simulink model "a1"  (Simulink 5.0)
settings: Solver=ode45  SolverMode=SingleTasking  StartTime=0.0  StopTime=1  RelTol=1e-4  AbsTol=1e-8
CloseFcn:
  | ;slview('closediagram',bdroot);
settings Model: LastModifiedBy=Âlue Phoenix  LimitDataPoints=off  BlockReductionOpt=off  BooleanDataType=off

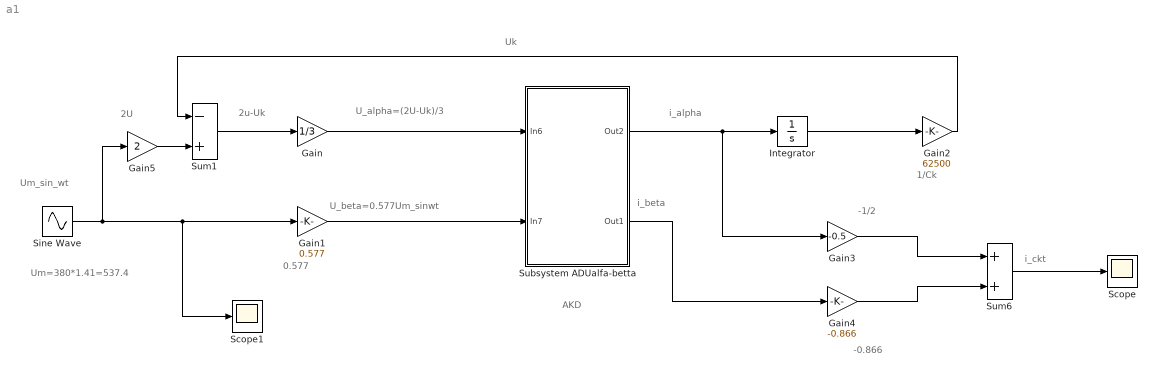
== system a1 ==
  note: U_alpha=(2U-Uk)/3
  note: Uk
  note: i_alpha
  note: i_beta
  note: 1/Ck
  note: -1/2
  note: -0.866
  note: i_ckt
  note: AKD
  note: Um_sin_wt
  note: Um=380*1.41=537.4
  note: 0.577
  note: 2U
  note: U_beta=0.577Um_sinwt
  note: 2u-Uk
  Gain : Gain  Gain=1/3  SaturateOnIntegerOverflow=on
  Gain1 : Gain  Gain=0.577  SaturateOnIntegerOverflow=on
  Gain2 : Gain  Gain=62500  SaturateOnIntegerOverflow=on
  Gain3 : Gain  Gain=-0.5  SaturateOnIntegerOverflow=on
  Gain4 : Gain  Gain=-0.866  SaturateOnIntegerOverflow=on
  Gain5 : Gain  Gain=2  SaturateOnIntegerOverflow=on
  Integrator : Integrator
  Scope : Scope
      settings: SaveName=ScopeData2
  Scope1 : Scope
      settings: SaveName=ScopeData3
  Sine Wave : Sin  Amplitude=537.4  Frequency=314  SampleTime=0
  Subsystem ADUalfa-betta : Subsystem
  Sum1 : Sum  Inputs=-+  SaturateOnIntegerOverflow=on  InputSameDT=on
  Sum6 : Sum  SaturateOnIntegerOverflow=on  InputSameDT=on
  wires:
  Sum1/1 -> Gain/1
  Gain/1 -> Subsystem ADUalfa-betta/1(In6)
  Gain1/1 -> Subsystem ADUalfa-betta/2(In7)
  Sine Wave/1 -> Gain1/1, Scope1/1, Gain5/1
  Subsystem ADUalfa-betta/1(Out2) -> Integrator/1, Gain3/1
  Integrator/1 -> Gain2/1
  Gain3/1 -> Sum6/1
  Gain4/1 -> Sum6/2
  Subsystem ADUalfa-betta/2(Out1) -> Gain4/1
  Gain2/1 -> Sum1/1
  Sum6/1 -> Scope/1
  Gain5/1 -> Sum1/2

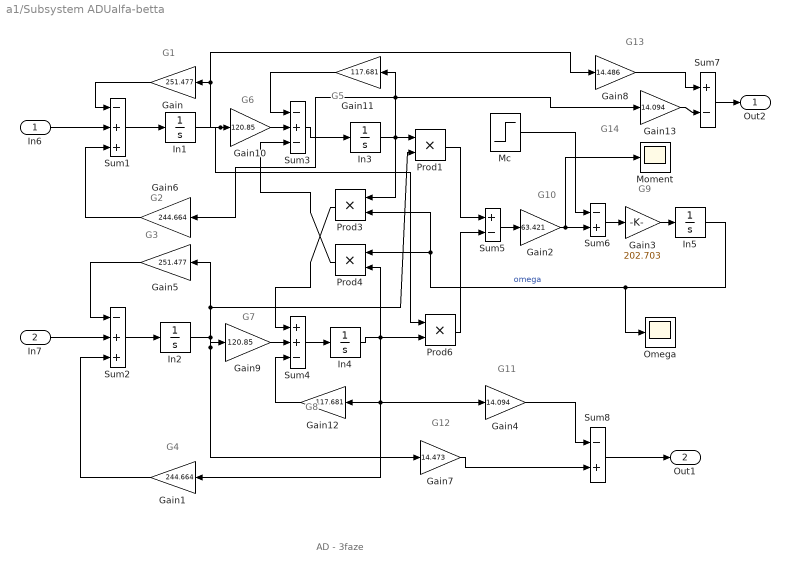
== system a1/Subsystem ADUalfa-betta ==
  note: G1
  note: G2
  note: G3
  note: G4
  note: G10
  note: G9
  note: G6
  note: G7
  note: G8
  note: G5
  note: AD - 3faze
  note: G14
  note: G12
  note: G13
  note: G11
  In6 : Inport
  In7 : Inport  Port=2
  "  Prod1" : Product  SaturateOnIntegerOverflow=on  InputSameDT=on
  Gain : Gain  Orientation=left  Gain=251.477  SaturateOnIntegerOverflow=on
  Gain1 : Gain  Orientation=left  Gain=244.664  SaturateOnIntegerOverflow=on
  Gain10 : Gain  Gain=120.85  SaturateOnIntegerOverflow=on
  Gain11 : Gain  Orientation=left  Gain=117.681  SaturateOnIntegerOverflow=on
  Gain12 : Gain  Orientation=left  Gain=117.681  SaturateOnIntegerOverflow=on
  Gain13 : Gain  Gain=14.094  SaturateOnIntegerOverflow=on
  Gain2 : Gain  Gain=63.421  SaturateOnIntegerOverflow=on
  Gain3 : Gain  Gain=202.703  SaturateOnIntegerOverflow=on
  Gain4 : Gain  Gain=14.094  SaturateOnIntegerOverflow=on
  Gain5 : Gain  Orientation=left  Gain=251.477  SaturateOnIntegerOverflow=on
  Gain6 : Gain  Orientation=left  Gain=244.664  SaturateOnIntegerOverflow=on
  Gain7 : Gain  Gain=14.473  SaturateOnIntegerOverflow=on
  Gain8 : Gain  Gain=14.486  SaturateOnIntegerOverflow=on
  Gain9 : Gain  Gain=120.85  SaturateOnIntegerOverflow=on
  In{1..5} (5 alike) : Integrator
  Mc : Step  Time=0.1  Before=0.0  After=17  SampleTime=0
  Moment : Scope
      settings: TickLabels=on  TimeRange=1  YMin=-10  YMax=20  DataFormat=Array
  Omega : Scope
      settings: TickLabels=on  TimeRange=0.5  YMin=0  YMax=1000  DataFormat=Array
  Prod3 : Product  Orientation=left  SaturateOnIntegerOverflow=on  InputSameDT=on
  Prod4 : Product  Orientation=left  SaturateOnIntegerOverflow=on  InputSameDT=on
  Prod6 : Product  SaturateOnIntegerOverflow=on  InputSameDT=on
  Sum1 : Sum  Inputs=-++  SaturateOnIntegerOverflow=on  InputSameDT=on
  Sum2 : Sum  Inputs=-++  SaturateOnIntegerOverflow=on  InputSameDT=on
  Sum3 : Sum  Inputs=-+-  SaturateOnIntegerOverflow=on  InputSameDT=on
  Sum4 : Sum  Inputs=++-  SaturateOnIntegerOverflow=on  InputSameDT=on
  Sum5 : Sum  Inputs=+-  SaturateOnIntegerOverflow=on  InputSameDT=on
  Sum6 : Sum  Inputs=-+  SaturateOnIntegerOverflow=on  InputSameDT=on
  Sum7 : Sum  Inputs=+-  SaturateOnIntegerOverflow=on  InputSameDT=on
  Sum8 : Sum  Inputs=-+  SaturateOnIntegerOverflow=on  InputSameDT=on
  Out2 : Outport
  Out1 : Outport  Port=2
  wires:
  Gain/1 -> Sum1/1
  Sum2/1 -> In2/1
  In4/1 -> Prod4/2, Prod6/2, Gain1/1, Gain12/1, Gain4/1
  In3/1 -> Prod3/1, "  Prod1"/1, Gain6/1, Gain11/1, Gain13/1
  Prod6/1 -> Sum5/2
  Sum6/1 -> Gain3/1
  Gain3/1 -> In5/1
  Mc/1 -> Sum6/1
  "  Prod1"/1 -> Sum5/1
  Sum3/1 -> In3/1
  Sum5/1 -> Gain2/1
  Sum1/1 -> In1/1
  In2/1 -> "  Prod1"/2, Gain5/1, Gain9/1, Gain7/1
  In1/1 -> Gain10/1, Gain/1, Gain8/1, Prod6/1
  Gain10/1 -> Sum3/2
  Gain9/1 -> Sum4/2
  Gain5/1 -> Sum2/1
  Prod4/1 -> Sum3/3
  Prod3/1 -> Sum4/1
  Gain2/1 -> Sum6/2, Moment/1
  Gain11/1 -> Sum3/1
  Gain12/1 -> Sum4/3
  In5/1 -> Prod3/2, Prod4/1, Omega/1  "omega"
  Sum4/1 -> In4/1
  Gain7/1 -> Sum8/2
  Gain4/1 -> Sum8/1
  Gain6/1 -> Sum1/3
  Gain1/1 -> Sum2/3
  In7/1 -> Sum2/2
  Gain8/1 -> Sum7/1
  Gain13/1 -> Sum7/2
  In6/1 -> Sum1/2
  Sum8/1 -> Out1/1
  Sum7/1 -> Out2/1
